simulink model "Simulink_copter_propeller_angle"  (R2016b)
settings: Solver=ode4  StartTime=0.0  StopTime=10.0  FixedStep=10e-3  RelTol=1e-3
InitFcn:
  | m = 1
  | L = 2
  | g = 9.81
  | c = 0.5
settings Model: Creator=bits  LastModifiedBy=bits

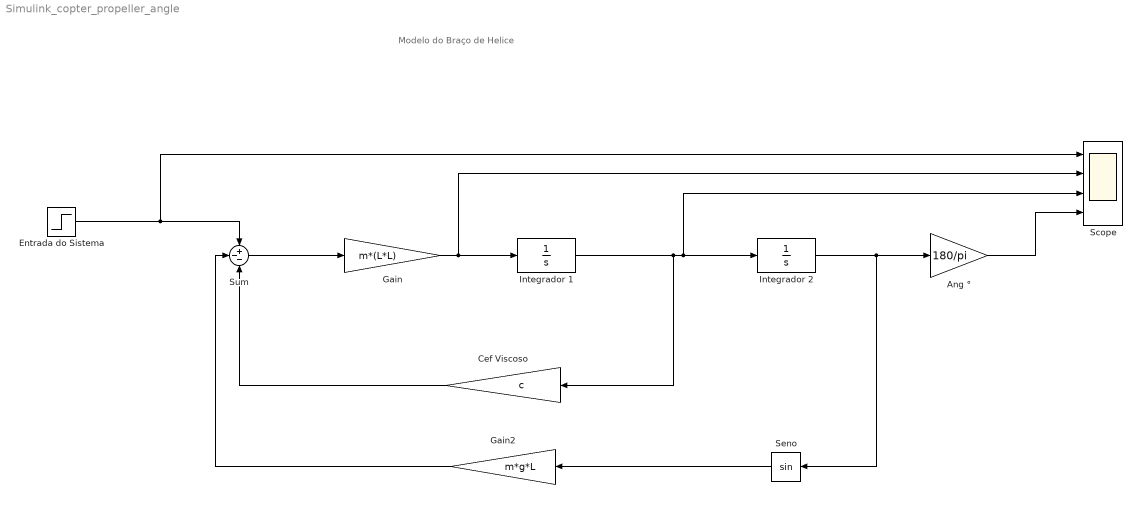
== system Simulink_copter_propeller_angle ==
  note: Modelo do Braço de Helice
  Ang ° : Gain  Gain=180/pi
  Cef Viscoso : Gain  Gain=c
  Entrada do Sistema : Step  After=15  SampleTime=0
  Gain : Gain  Gain=m*(L*L)
  Gain2 : Gain  Gain=m*g*L
  Integrador 1 : TransferFcn  Denominator=[1 0]
  Integrador 2 : TransferFcn  Denominator=[1 0]
  Scope : Scope  NumInputPorts=4
  Seno : Trigonometry
  Sum : Sum  Inputs=+--
  wires:
  Entrada do Sistema/1 -> Sum/1, Scope/1
  Integrador 2/1 -> Ang °/1, Seno/1
  Integrador 1/1 -> Scope/3, Integrador 2/1, Cef Viscoso/1
  Gain/1 -> Scope/2, Integrador 1/1
  Sum/1 -> Gain/1
  Cef Viscoso/1 -> Sum/3
  Gain2/1 -> Sum/2
  Seno/1 -> Gain2/1
  Ang °/1 -> Scope/4
